simulink model "lpv_model"  (R2019a)
settings: Solver=VariableStepAuto  StartTime=0.0  StopTime=10.0  RelTol=1e-3
libraries: simulink x2, shared6dof x1
settings Model: Creator=marin  LastModifiedBy=marin

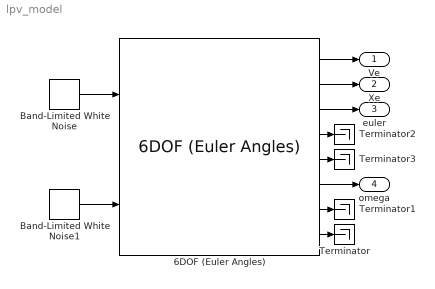
== system lpv_model ==
  6DOF (Euler Angles) : shared6dof/6DOF (Euler Angles)  units=Metric (MKS)  mtype=Fixed  rep=Euler Angles  xme_0=[0 0 0]  Vm_0=[0 0 0]  eul_0=[0 0 0]  pm_0=[0 0 0]  mass_0=1.0  mass_e=0.5  mass_f=2.0  inertia=eye(3)  inertia_e=eye(3)  inertia_f=2*eye(3)  k_quat=1.0  vre_flag=on  abi_flag=off  aMode=0  xme_statename=''  Vm_statename=''  eul_statename=''  quat_statename=''  pm_statename=''  mass_statename=''
      settings: SourceProductBaseCode=AE
  Band-Limited White Noise : simulink/Sources/Band-Limited White Noise  Cov=[1, 1, 1]'  Ts=1  seed=[2, 33, 41]
  Band-Limited White Noise1 : simulink/Sources/Band-Limited White Noise  Cov=[1, 1, 1]'  Ts=1  seed=[23, 3, 41]
  Terminator{,1..3} (4 alike) : Terminator
  Ve : Outport
  Xe : Outport  Port=2
  euler : Outport  Port=3
  omega : Outport  Port=4
  wires:
  Band-Limited White Noise1/1 -> 6DOF (Euler Angles)/2
  Band-Limited White Noise/1 -> 6DOF (Euler Angles)/1
  6DOF (Euler Angles)/2 -> Xe/1
  6DOF (Euler Angles)/1 -> Ve/1
  6DOF (Euler Angles)/8 -> Terminator/1
  6DOF (Euler Angles)/7 -> Terminator1/1
  6DOF (Euler Angles)/6 -> omega/1
  6DOF (Euler Angles)/5 -> Terminator3/1
  6DOF (Euler Angles)/3 -> euler/1
  6DOF (Euler Angles)/4 -> Terminator2/1
